simulink model "MultirotorModel"  (R2024b)
settings: Solver=VariableStepAuto  StartTime=0.0  StopTime=simTime  FixedStep=0.001  RelTol=1e-3  EnableMultiTasking=on
undefined symbols (not defined in the file): baseMission, bird_cycle, bird_end, bird_start, Controller, ctrl_mass, ctrl_thrust_perturbation_param, DiscIntNeverNeededParam, Dz, Earth, Gravity, initialConditions, Iz, mass_param, Nz, Pz, startFlightTime, UAVSampleTime, Vehicle, WGS84
libraries: slpidlib x10, uavalgslib x6, simulink x3, sharedutil x2, aerolibconvert2 x2, aerolibtransform2 x2, robotcorelib x1, uavutilslib x1, shared6dof x1, aerolibasang x1, sensorinslib x1
(part 1 of 3)
settings Model: DataDictionary=uavPackageDeliveryDataDict.sldd  ModifiedByFormat=The MathWorks, Inc.  SimulationMode=accelerator  PacingRate=3  Creator=The MathWorks, Inc.  LastModifiedBy=The MathWorks, Inc.
settings SolverCC: AlgebraicLoopSolver=TrustRegion  AutoInsertRateTranBlk=on  MaxZcPerStep=1
settings DataIOCC: LimitDataPoints=on  SaveOutput=off  SaveTime=off  ReturnWorkspaceOutputs=off
settings OptimizationCC: ReuseModelBlockBuffer=off  LifeSpan=inf
settings DebuggingCC: RTPrefix=none  SignalInfNanChecking=error  SignalRangeChecking=error  CheckMatrixSingularityMsg=error  ParameterPrecisionLossMsg=none  AllowSymbolicDim=off  SFUnexpectedBacktrackingDiag=warning  SFNoUnconditionalDefaultTransitionDiag=warning  SFExecutionAtInitializationDiag=none  ArithmeticOperatorsInVariantConditions=warning
settings ModelReferenceCC: EnableRefExpFcnMdlSchedulingChecks=on  PropagateSignalLabelsOutOfModel=off
settings SFSimCC: SimUseLocalCustomCode=off  CustomCodeUndefinedFunction=UseInterfaceOnly
settings RTWCC: RTWUseLocalCustomCode=off  GPUComputeCapability=3.5  DLArmComputeVersion=19.05
settings CodeAppCC: StateflowObjectComments=on
settings GRTTargetCC: TargetLangStandard=C89/C90 (ANSI)
settings ConfigComp: CovMetricSettings=dw  CovSaveCumulativeToWorkspaceVar=on  CovSaveSingleToWorkspaceVar=on  CovExternalEMLEnable=off

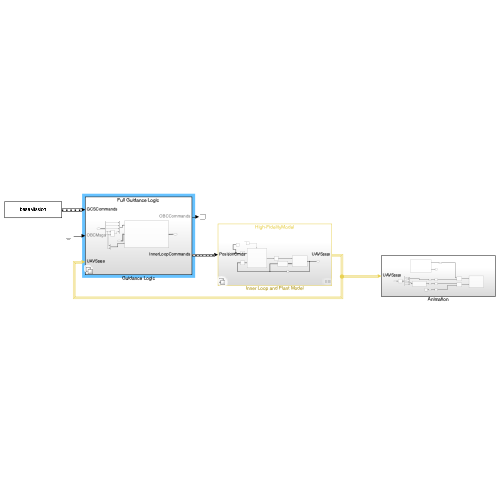
[thumbnail: Simulink's stored preview of the top-level diagram]
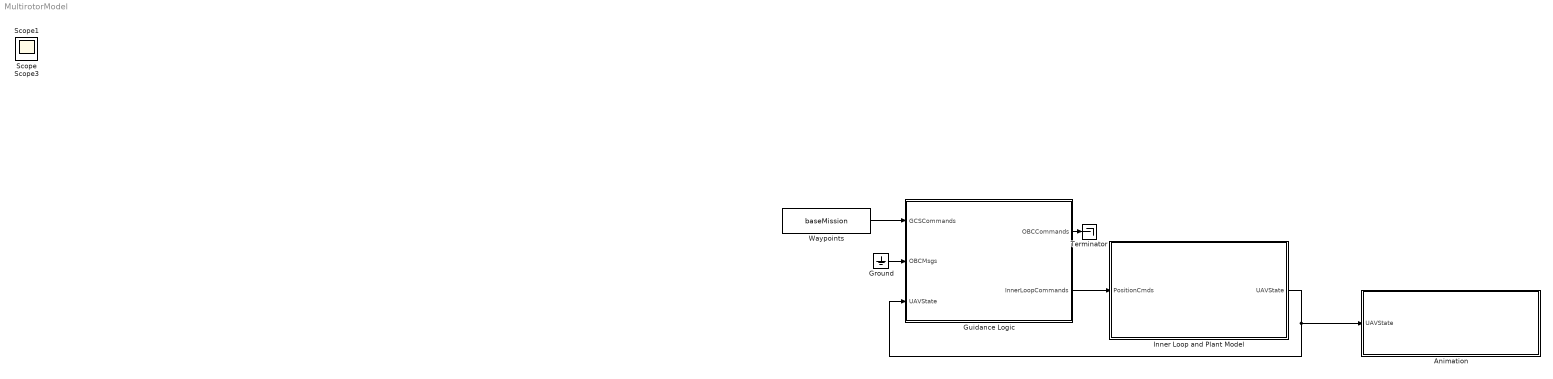
== system MultirotorModel ==
  Animation : Subsystem
  Ground : Ground
  Guidance Logic : Subsystem  Variant=on
  Inner Loop and Plant Model : Subsystem  Variant=on
  Terminator : Terminator
  Waypoints : Constant  Value=baseMission  OutDataTypeStr=Bus: uavPathManagerBus  SampleTime=-1
  Scope : Scope
  Scope1 : Scope
  Scope3 : Scope
  wires:
  Guidance Logic/2(InnerLoopCommands) -> Inner Loop and Plant Model/1(PositionCmds)
  Guidance Logic/1(OBCCommands) -> Terminator/1
  Ground/1 -> Guidance Logic/2(OBCMsgs)
  Waypoints/1 -> Guidance Logic/1(GCSCommands)
  Inner Loop and Plant Model/1(UAVState) -> Guidance Logic/3(UAVState), Animation/1(UAVState)

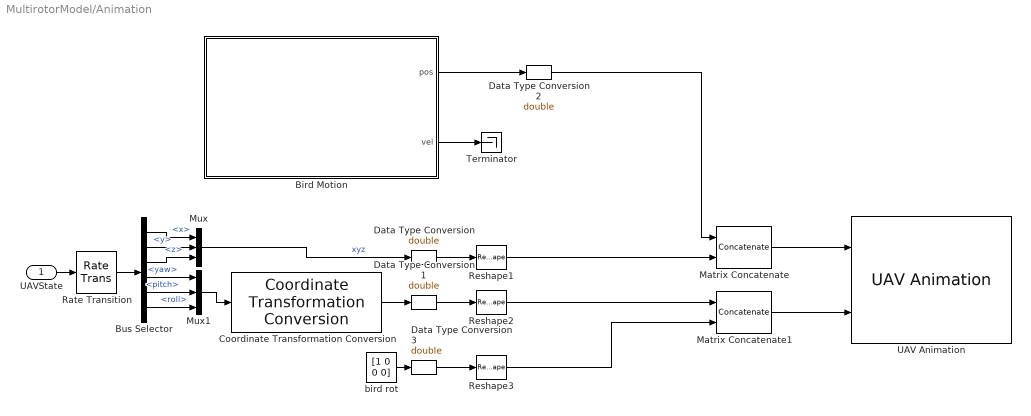
== system MultirotorModel/Animation ==
  UAVState : Inport
  Bird Motion : Subsystem
  Bus Selector : BusSelector  OutputSignals=pos_vel.x,pos_vel.y,pos_vel.z,attitude.yaw,attitude.pitch,attitude.roll
  Coordinate Transformation Conversion : robotcorelib/Coordinate Transformation Conversion  InputRepresentation=Euler Angles  InputEulerSequence=ZYX  ShowTrVecInputPort=on  OutputRepresentation=Quaternion  OutputEulerSequence=ZYX  ShowTrVecOutputPort=on  SimulateUsing=Code generation
  Data Type Conversion{,1..3} (4 alike) : DataTypeConversion  OutDataTypeStr=double  SaturateOnIntegerOverflow=off  RndMeth=Floor
  Matrix Concatenate : Concatenate  Mode=Multidimensional array
  Matrix Concatenate1 : Concatenate  Mode=Multidimensional array
  Mux : Mux  Inputs=3
  Mux1 : Mux  Inputs=3
  Rate Transition : RateTransition  OutPortSampleTime=UAVSampleTime*200
  Reshape1 : Reshape  OutputDimensionality=Row vector (2-D)
  Reshape2 : Reshape  OutputDimensionality=Row vector (2-D)
  Reshape3 : Reshape  OutputDimensionality=Row vector (2-D)
  Terminator : Terminator
  UAV Animation : uavutilslib/UAV Animation  NumUAV=2  DynamicUAVConfig=off  UAVType=Multirotor  UAVSize=1  UAVColor=[1 0 0]  UAVTrajectoryAlpha=1  InertialZDirection=Down  RotationFormat=Quaternion  DrawMarkers=off  SampleTime=UAVSampleTime*200
  bird rot : Constant  Value=[1 0 0 0]
  wires:
  Bus Selector/1 -> Mux/1  "<x>"
  Bus Selector/2 -> Mux/2  "<y>"
  Coordinate Transformation Conversion/1 -> Data Type Conversion1/1
  Rate Transition/1 -> Bus Selector/1
  Mux/1 -> Data Type Conversion/1  "xyz"
  UAVState/1 -> Rate Transition/1
  Bus Selector/6 -> Mux1/3  "<roll>"
  Bus Selector/4 -> Mux1/1  "<yaw>"
  Bus Selector/3 -> Mux/3  "<z>"
  Mux1/1 -> Coordinate Transformation Conversion/1
  Bus Selector/5 -> Mux1/2  "<pitch>"
  bird rot/1 -> Data Type Conversion3/1
  Data Type Conversion/1 -> Reshape1/1
  Data Type Conversion1/1 -> Reshape2/1
  Data Type Conversion3/1 -> Reshape3/1
  Data Type Conversion2/1 -> Matrix Concatenate/1
  Reshape1/1 -> Matrix Concatenate/2
  Matrix Concatenate/1 -> UAV Animation/1
  Reshape2/1 -> Matrix Concatenate1/1
  Reshape3/1 -> Matrix Concatenate1/2
  Matrix Concatenate1/1 -> UAV Animation/2
  Bird Motion/1(pos) -> Data Type Conversion2/1
  Bird Motion/2(vel) -> Terminator/1

== system MultirotorModel/Guidance Logic ==
  GCSCommands : Inport
  OBCMsgs : Inport  Port=2
  UAVState : Inport  Port=3
  Full Guidance Logic : Subsystem  TreatAsAtomicUnit=on  VariantControl=guidanceType==1
  Obstacle Avoidance : Subsystem  TreatAsAtomicUnit=on  SystemSampleTime=0.005*4  VariantControl=guidanceType ==2
  Obstacle Avoidance3D : Subsystem  TreatAsAtomicUnit=on  SystemSampleTime=0.005*4  VariantControl=guidanceType ==3
  OBCCommands : Outport  SampleTime=0.005  BusOutputAsStruct=on
  InnerLoopCommands : Outport  Port=2

== system MultirotorModel/Inner Loop and Plant Model ==
  PositionCmds : Inport
  High-FidelityModel : Subsystem  VariantControl=plantModelFi==1
  Low-FidelityModel : Subsystem  VariantControl=plantModelFi ==0
  UAVState : Outport

== system MultirotorModel/Animation/Bird Motion ==
  BirdMotion : MATLAB Function  TreatAsAtomicUnit=on
  Constant : Constant  Value=0.02
  Constant1 : Constant  Value=bird_start
  Constant2 : Constant  Value=bird_end
  Constant3 : Constant  Value=bird_cycle
  Demux : Demux  Outputs=6
  Mux : Mux  Inputs=3
  Mux1 : Mux  Inputs=3
  Reshape : Reshape  OutputDimensionality=Row vector (2-D)
  Sum : Sum  Inputs=|++
  Unit Delay : UnitDelay  SampleTime=0.02  HasFrameUpgradeWarning=on
  pos : Outport
  vel : Outport  Port=2
  wires:
  Unit Delay/1 -> Sum/2, BirdMotion/1(t)
  Sum/1 -> Unit Delay/1
  Constant/1 -> Sum/1
  Constant1/1 -> BirdMotion/2(start_pt)
  Constant2/1 -> BirdMotion/3(end_pt)
  Constant3/1 -> BirdMotion/4(cycle_time)
  BirdMotion/1(out) -> Demux/1
  Demux/1 -> Mux/1
  Demux/2 -> Mux/2
  Demux/3 -> Mux/3
  Demux/4 -> Mux1/1
  Demux/5 -> Mux1/2
  Demux/6 -> Mux1/3
  Mux/1 -> Reshape/1
  Mux1/1 -> vel/1
  Reshape/1 -> pos/1

== system MultirotorModel/Guidance Logic/Full Guidance Logic ==
  UAVState : Inport
  GCSCommands : Inport  Port=2
  Atan2 : Trigonometry  Operator=atan2
  Bus Selector1 : BusSelector  OutputSignals=pos_vel.x,pos_vel.y,pos_vel.z,pos_vel.vy,pos_vel.vx
  DroneVel : Mux  Inputs=2
  Guidance Stateflow : Subsystem
  Mux : Mux
  InnerLoopCommands : Outport
  wires:
  Mux/1 -> Guidance Stateflow/1(Pose)
  Bus Selector1/5 -> DroneVel/1, Atan2/2  "<vx>"
  Guidance Stateflow/1(InnerLoopCommands) -> InnerLoopCommands/1
  Bus Selector1/4 -> Atan2/1, DroneVel/2  "<vy>"
  Bus Selector1/3 -> Mux/3  "<z>"
  Bus Selector1/2 -> Mux/2  "<y>"
  UAVState/1 -> Bus Selector1/1
  Atan2/1 -> Mux/4
  Bus Selector1/1 -> Mux/1  "<x>"
  GCSCommands/1 -> Guidance Stateflow/2(GCSCommands)
  DroneVel/1 -> Guidance Stateflow/3(DroneVel)

== system MultirotorModel/Guidance Logic/Obstacle Avoidance ==
  GCSCommands : Inport
  OBCMsgs : Inport  Port=2
  UAVState : Inport  Port=3
  Bus Selector : BusSelector  OutputSignals=pos_vel
  Compute InnerLoop Cmds : Subsystem  TreatAsAtomicUnit=on
  MATLAB Function : MATLAB Function  TreatAsAtomicUnit=on
  Selector : Selector  InputPortWidth=42  IndexOptions=Index vector (dialog)  Indices=[1 2]  OutputSizes=1
  Unit Delay1 : UnitDelay  InitialCondition=single(0)  SampleTime=-1  HasFrameUpgradeWarning=on
  InnerLoopCommands : Outport
  OBCCommands : Outport  Port=2  BusOutputAsStruct=on
  wires:
  GCSCommands/1 -> Selector/1
  Unit Delay1/1 -> MATLAB Function/2(Steer)
  UAVState/1 -> Compute InnerLoop Cmds/2(UAVState), Bus Selector/1
  Bus Selector/1 -> MATLAB Function/3(UAVState)  "<pos_vel>"
  Selector/1 -> OBCCommands/1, MATLAB Function/1(mission)
  Compute InnerLoop Cmds/1(InnerLoopCmds) -> InnerLoopCommands/1
  MATLAB Function/1(y) -> Compute InnerLoop Cmds/1(GCSCmds)
  OBCMsgs/1 -> Unit Delay1/1

== system MultirotorModel/Guidance Logic/Obstacle Avoidance3D ==
  GCSCommands : Inport
  OBCMsgs : Inport  Port=2
  UAVState : Inport  Port=3
  Bus Selector : BusSelector  OutputSignals=pos_vel
  Compute InnerLoop Cmds : Subsystem  TreatAsAtomicUnit=on
  MATLAB Function : MATLAB Function  TreatAsAtomicUnit=on
  Selector : Selector  InputPortWidth=42  IndexOptions=Index vector (dialog)  Indices=[1 2]  OutputSizes=1
  Unit Delay1 : UnitDelay  InitialCondition=single(0)  SampleTime=-1  HasFrameUpgradeWarning=on
  InnerLoopCommands : Outport
  OBCCommands : Outport  Port=2  BusOutputAsStruct=on
  wires:
  MATLAB Function/1(y) -> Compute InnerLoop Cmds/1(GCSCmds)
  Unit Delay1/1 -> MATLAB Function/2(Steer)
  Selector/1 -> MATLAB Function/1(mission), OBCCommands/1
  Bus Selector/1 -> MATLAB Function/3(UAVState)  "<pos_vel>"
  GCSCommands/1 -> Selector/1
  OBCMsgs/1 -> Unit Delay1/1
  MATLAB Function/2(DTD) -> Compute InnerLoop Cmds/2(DTD)
  Compute InnerLoop Cmds/1(InnerLoopCmds) -> InnerLoopCommands/1
  UAVState/1 -> Bus Selector/1, Compute InnerLoop Cmds/4(UAVState)
  MATLAB Function/3(needHover) -> Compute InnerLoop Cmds/3(needHover)

== system MultirotorModel/Inner Loop and Plant Model/High-FidelityModel ==
  note: To be replaced with a signal from the GCS to "Start Mission"
  PositionCmds : Inport
  Control System : Subsystem  TreatAsAtomicUnit=on  SystemSampleTime=UAVSampleTime
  Environment : Subsystem  TreatAsAtomicUnit=on  VariantControl=VSS_ENVIRONMENT_VARIABLE
  Memory1 : Memory  InheritSampleTime=on  LinearizeMemory=on  LinearizeAsDelay=on
  Plant Model : Subsystem  TreatAsAtomicUnit=on
  Rate Transition : RateTransition
  Rate Transition1 : RateTransition  OutPortSampleTime=UAVSampleTime
  Rate Transition2 : RateTransition  OutPortSampleTime=UAVSampleTime
  Scope : Scope
  Step : Step  Time=startFlightTime  SampleTime=UAVSampleTime
  UAVState : Outport  OutDataTypeStr=Bus: uavStateBus
  wires:
  PositionCmds/1 -> Scope/1, Rate Transition1/1
  Control System/1(ActuatorCmds) -> Rate Transition/1  "motors"
  Environment/1(Environment) -> Plant Model/2(Environment)
  Memory1/1 -> Environment/1(States), Rate Transition2/1
  Plant Model/1(UAVState) -> UAVState/1, Memory1/1
  Step/1 -> Control System/Enable
  Rate Transition/1 -> Plant Model/1(Actuators)
  Rate Transition1/1 -> Control System/1(PositionCmd)
  Rate Transition2/1 -> Control System/2(UAVState)

== system MultirotorModel/Inner Loop and Plant Model/Low-FidelityModel ==
  PositionCmds : Inport
  Assemble UAV State Bus : Subsystem
  Bus Creator1 : BusCreator  Inputs=1  OutDataTypeStr=Bus: uavGuidanceEnvironmentBus  NonVirtualBus=on
  Constant : Constant  Value=Gravity  OutDataTypeStr=single
      settings: AttributesFormatString=%<Value>
  Position and Acceleration Control : Subsystem
  Quadrotor Plant : uavalgslib/Guidance Model  ModelType=MultirotorGuidance  SpecifiedDataType=single  SimulateUsing=Code generation  InitialWorldPositionMultirotor=[-186; -105; 0]  InitialWorldVelocityMultirotor=[0; 0; 0]  InitialEulerZYXMultirotor=[0; 0; 0]  InitialBodyAngularRateRPYMultirotor=[0; 0; 0]  InitialThrustMultirotor=0  InitialNorthFixedWing=0  InitialEastFixedWing=0  InitialHeightFixedWing=0  InitialAirSpeedFixedWing=0  InitialHeadingAngleFixedWing=0  InitialFlightPathAngleFixedWing=0  InitialRollAngleFixedWing=0  InitialRollAngleRateFixedWing=0  PDRollMultirotor=[3402.97,116.67]  PDPitchMultirotor=[3402.97, 116.67]  PYawRateMultirotor=1950  PThrustMultirotor=39  MassMultirotor=0.1  PHeightFixedWing=3.9  PHeadingAngleFixedWing=3.9  PFlightPathAngleFixedWing=39  PDRollFixedWing=[3402.97, 116.67]  PAirSpeedFixedWing=1  FlightPathAngleLimitsFixedWing=[-pi/2, pi/2]  StateBusName='uavGuidanceStateBus'  ControlBusName='uavGuidanceControlBus'  EnvironmentBusName='uavGuidanceEnvironmentBus'  DataType=single
  Rate Transition1 : RateTransition  OutPortSampleTime=UAVSampleTime
  Rate Transition2 : RateTransition  OutPortSampleTime=UAVSampleTime
  UAVState : Outport  OutDataTypeStr=Bus: uavStateBus
  wires:
  Constant/1 -> Bus Creator1/1  "Gravity"
  Bus Creator1/1 -> Quadrotor Plant/2
  Position and Acceleration Control/1(Control Signal) -> Rate Transition2/1
  Quadrotor Plant/1 -> Rate Transition1/1
  Rate Transition2/1 -> Quadrotor Plant/1
  PositionCmds/1 -> Position and Acceleration Control/2(PositionCmd)
  Rate Transition1/1 -> Position and Acceleration Control/1(QuadRotorState), Assemble UAV State Bus/1(State)
  Assemble UAV State Bus/1(UAVState) -> UAVState/1

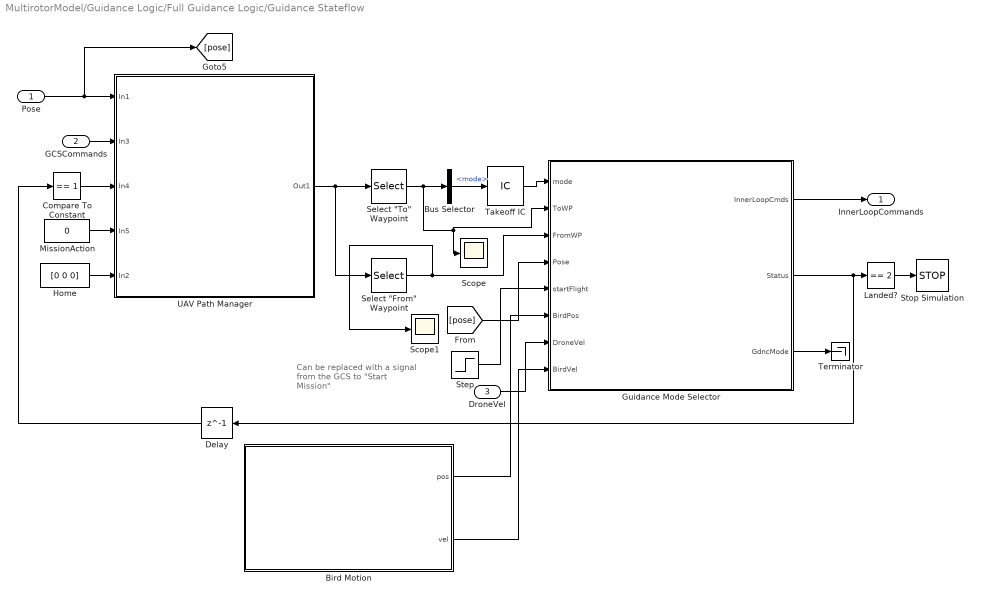
== system MultirotorModel/Guidance Logic/Full Guidance Logic/Guidance Stateflow ==
  note: Can be replaced with a signal from the GCS to "Start Mission"
  Pose : Inport
  GCSCommands : Inport  Port=2
  DroneVel : Inport  Port=3
  Bird Motion : Subsystem
  Bus Selector : BusSelector  OutputSignals=mode
  Compare To Constant : simulink/Logic and Bit Operations/Compare To Constant  relop===  const=1  OutDataTypeStr=boolean
  Delay : Delay  DelayLength=1  InitialCondition=0
  Guidance Mode Selector : Stateflow chart  TreatAsAtomicUnit=on
  Home : Constant  Value=[0 0 0]  OutDataTypeStr=single
  Landed? : simulink/Logic and Bit Operations/Compare To Constant  relop===  const=2  OutDataTypeStr=boolean
  MissionAction : Constant  Value=0  OutDataTypeStr=uint8
  Scope : Scope
  Scope1 : Scope
  "Select \"From\" Waypoint" : Selector  InputPortWidth=2  IndexOptions=Index vector (dialog)  Indices=2  OutputSizes=1
  "Select \"To\" Waypoint" : Selector  InputPortWidth=2  IndexOptions=Index vector (dialog)  Indices=1  OutputSizes=1
  Step : Step  Time=startFlightTime  SampleTime=UAVSampleTime*4
  Stop Simulation : Stop
  Takeoff IC : InitialCondition
  Terminator : Terminator
  UAV Path Manager : Subsystem  AncestorBlock=uavalgslib/Path Manager  mask(Path Manager){UAVType=multirotor, LoiterRadius=25, dataType=single, inputBusName='uavPathManagerBus', SimulateUsing=Code generation}
      mask prompts: UAVType "uav:robotsluav:pathmanager:UAVType"; LoiterRadius "uav:robotsluav:pathmanager:LoiterRadius"; dataType "uav:robotsluav:pathmanager:DataType"; inputBusName "uav:robotsluav:pathmanager:InputBusName"; SimulateUsing "SystemBlock:MATLABSystem:SimulateUsing"
      mask help: uav:robotsluav:pathmanager:PathManagerDescription
      mask Help: eval('helpview(''uav'',''uavPathManager'')');
      mask TypeOptions UAVType: PathManagerSystemObject/UAVType
      mask Callback UAVType: uav.sluav.internal.pathmanager.mask.setLoiterParameter(gcb);
      mask TypeOptions LoiterRadius: PathManagerSystemObject/LoiterRadius
      mask Callback dataType:
      | if ~strcmp(get_param(gcb, 'dataType'), '<data type expression>')
      | 
      |     %create path manager bus
      |     uav.sluav.internal.pathmanager.mask.createUAVPathManagerBus(gcb);
      | 
      | end
      mask Callback inputBusName: uav.sluav.internal.pathmanager.mask.createUAVPathManagerBus(gcb);
      mask TypeOptions SimulateUsing: PathManagerSystemObject/SimulateUsing
      mask DialogControl UAVType Prompt: UAV type:
      mask DialogControl LoiterRadius Prompt: Loiter radius (m):
      mask DialogControl dataType Prompt: Data type:
      mask DialogControl inputBusName Prompt: Mission bus name:
      mask DialogControl SimulateUsing Prompt: Simulate using:
      mask Display:
      | port_label('input',1,'Pose')
      | port_label('input',2,'MissionData')
      | port_label('input',3,'isModeDone')
      | port_label('input',4,'MissionCmd')
      | port_label('input',5,'Home')
      | port_label('output',1,'MissionParams')
  InnerLoopCommands : Outport  OutDataTypeStr=Bus: innerLoopCmdsBus
  wires:
  Takeoff IC/1 -> Guidance Mode Selector/1(mode)
  Delay/1 -> Compare To Constant/1
  Guidance Mode Selector/2(Status) -> Delay/1, Landed?/1
  Guidance Mode Selector/1(InnerLoopCmds) -> InnerLoopCommands/1
  Pose/1 -> UAV Path Manager/1(In1), [pose]
  UAV Path Manager/1(Out1) -> "Select \"From\" Waypoint"/1, "Select \"To\" Waypoint"/1
  Bus Selector/1 -> Takeoff IC/1  "<mode>"
  [pose] -> Guidance Mode Selector/4(Pose)
  "Select \"To\" Waypoint"/1 -> Scope/1, Guidance Mode Selector/2(ToWP), Bus Selector/1
  "Select \"From\" Waypoint"/1 -> Scope1/1, Guidance Mode Selector/3(FromWP)
  Landed?/1 -> Stop Simulation/1
  Step/1 -> Guidance Mode Selector/5(startFlight)
  Guidance Mode Selector/3(GdncMode) -> Terminator/1
  Home/1 -> UAV Path Manager/5(In2)
  MissionAction/1 -> UAV Path Manager/4(In5)
  Compare To Constant/1 -> UAV Path Manager/3(In4)
  GCSCommands/1 -> UAV Path Manager/2(In3)
  Bird Motion/1(pos) -> Guidance Mode Selector/6(BirdPos)
  DroneVel/1 -> Guidance Mode Selector/7(DroneVel)
  Bird Motion/2(vel) -> Guidance Mode Selector/8(BirdVel)

== system MultirotorModel/Guidance Logic/Obstacle Avoidance/Compute InnerLoop Cmds ==
  GCSCmds : Inport
  UAVState : Inport  Port=2
  Atan2 : Trigonometry  Operator=atan2
  Bus Creator : BusCreator  Inputs=3  OutDataTypeStr=Bus: innerLoopCmdsBus  NonVirtualBus=on
  Bus Selector1 : BusSelector  OutputSignals=pos_vel.x,pos_vel.y,pos_vel.z,pos_vel.vy,pos_vel.vx
  Lookahead Distance : Constant  Value=5  OutDataTypeStr=single
  Mux : Mux
  Scope : Scope
  Scope1 : Scope
  Terminator : Terminator
  Waypoint Follower : uavalgslib/Waypoint Follower  UAVType=multirotor  StartFrom=first  TransitionRadiusSource=internal  TransitionRadius=0.5  MinLookaheadDistance=0.1  HoverAtLastWaypoint=off  YawInput=on  ShowCrossTrackErrorOutput=on  ShowStatusOutput=on  SimulateUsing=Code generation
  InnerLoopCmds : Outport  OutDataTypeStr=Bus: innerLoopCmdsBus
  wires:
  Atan2/1 -> Mux/4
  Lookahead Distance/1 -> Waypoint Follower/3
  UAVState/1 -> Bus Selector1/1
  Bus Selector1/2 -> Mux/2  "<y>"
  Bus Selector1/1 -> Mux/1  "<x>"
  Bus Selector1/4 -> Atan2/1  "<vy>"
  Mux/1 -> Waypoint Follower/1
  Bus Selector1/5 -> Atan2/2  "<vx>"
  Bus Selector1/3 -> Mux/3  "<z>"
  Bus Creator/1 -> InnerLoopCmds/1
  Waypoint Follower/1 -> Bus Creator/1  "LAP"
  Waypoint Follower/2 -> Bus Creator/2  "HeadingCmd"
  Waypoint Follower/3 -> Bus Creator/3  "YawCmd"
  GCSCmds/1 -> Waypoint Follower/2
  Waypoint Follower/5 -> Scope/1
  Waypoint Follower/4 -> Terminator/1
  Waypoint Follower/6 -> Scope1/1

== system MultirotorModel/Guidance Logic/Obstacle Avoidance3D/Compute InnerLoop Cmds ==
  GCSCmds : Inport
  DTD : Inport  Port=2
  needHover : Inport  Port=3
  UAVState : Inport  Port=4
  FollowWaypoints : Subsystem
  GCSCmds1 : InportShadow
  GCSCmds2 : InportShadow
  Hover : Subsystem
  Landing : Subsystem
  Switch1 : Switch  Threshold=5  SaturateOnIntegerOverflow=off  InputSameDT=off
  Switch2 : Switch  Criteria=u2 ~= 0  Threshold=5  SaturateOnIntegerOverflow=off  InputSameDT=off
  UAVState1 : InportShadow  Port=4
  InnerLoopCmds : Outport  OutDataTypeStr=Bus: innerLoopCmdsBus
  wires:
  Switch2/1 -> InnerLoopCmds/1
  GCSCmds2/1 -> Hover/1(In1)
  UAVState1/1 -> Landing/2(UAVState1)
  Hover/1(Out1) -> Switch2/1
  Landing/1(InnerLoopCmds1) -> Switch1/3
  Switch1/1 -> Switch2/3
  GCSCmds1/1 -> Landing/1(GCSCmds)
  FollowWaypoints/1(InnerLoopCmds) -> Switch1/1
  DTD/1 -> Switch1/2
  UAVState/1 -> FollowWaypoints/1(UAVState)
  GCSCmds/1 -> FollowWaypoints/2(GCSCmds)
  needHover/1 -> Switch2/2

== system MultirotorModel/Inner Loop and Plant Model/High-FidelityModel/Control System ==
  PositionCmd : Inport
  UAVState : Inport  Port=2  BusOutputAsStruct=on
  Enable : EnablePort  StatesWhenEnabling=reset
  Controller : Subsystem
  ActuatorCmds : Outport  VectorParamsAs1DForOutWhenUnconnected=off
  wires:
  Controller/1(motors_refout) -> ActuatorCmds/1
  UAVState/1 -> Controller/2(UAVState)
  PositionCmd/1 -> Controller/1(PositionCmd)

== system MultirotorModel/Inner Loop and Plant Model/High-FidelityModel/Environment ==
  States : Inport
  Bus Creator : BusCreator  Inputs=3  OutDataTypeStr=Bus: EnvironmentBus  NonVirtualBus=on
  Bus Creator1 : BusCreator  Inputs=4  OutDataTypeStr=Bus: AtmosphereBus  NonVirtualBus=on
  Bus Selector : BusSelector  OutputSignals=gps.lat,gps.lon,gps.alt
  Constant : Constant  Value=288.08
  Constant1 : Constant  Value=340.25
  Constant2 : Constant  Value=1.012*10^5
  Constant3 : Constant  Value=1.224
  Gain : Gain  Gain=1/1e7  OutDataTypeStr=double
  Gain1 : Gain  Gain=1/1e7  OutDataTypeStr=double
  Gain2 : Gain  Gain=1/-1e3  OutDataTypeStr=double
  Magnetic feild : Constant  Value=[19080, -1276, 50282]
  Mux : Mux  Inputs=3
  "WGS84 Gravity Model  " : GravityWGS84  action=None
  Environment : Outport  VectorParamsAs1DForOutWhenUnconnected=off
  wires:
  States/1 -> Bus Selector/1  "StatesLog"
  Bus Creator/1 -> Environment/1
  Bus Creator1/1 -> Bus Creator/2  "AtmosphereBus"
  "WGS84 Gravity Model  "/1 -> Bus Creator/1  "Gravity_ned"
  Mux/1 -> "WGS84 Gravity Model  "/1
  Gain/1 -> Mux/1
  Bus Selector/1 -> Gain/1  "<lat>"
  Bus Selector/2 -> Gain1/1  "<lon>"
  Gain1/1 -> Mux/2
  Bus Selector/3 -> Gain2/1  "<alt>"
  Gain2/1 -> Mux/3
  Magnetic feild/1 -> Bus Creator/3  "MagneticField_ned"
  Constant/1 -> Bus Creator1/1  "air_temp"
  Constant1/1 -> Bus Creator1/2  "speed_sound"
  Constant2/1 -> Bus Creator1/3  "pressure"
  Constant3/1 -> Bus Creator1/4  "air_density"

== system MultirotorModel/Inner Loop and Plant Model/High-FidelityModel/Plant Model ==
  Actuators : Inport
  Environment : Inport  Port=2
  6DOF (Quaternion) : shared6dof/6DOF (Euler Angles)  units=Metric (MKS)  mtype=Fixed  rep=Euler Angles  xme_0=initialConditions.posNED + [0 0 -1]  Vm_0=[0 0 0]  eul_0=[0,0,0]  pm_0=[0,0,0]  mass_0=mass_param  mass_e=0.5  mass_f=2.0  inertia=Vehicle.Airframe.inertia  inertia_e=eye(3)  inertia_f=2*eye(3)  k_quat=Vehicle.SixDOF.quatGain  vre_flag=on  abi_flag=on  aMode=aMode  xme_statename=''  Vm_statename=''  eul_statename=''  quat_statename=''  pm_statename=''  mass_statename=''
  AC model : Subsystem
  Bus setup : Subsystem
  IMU Drift : FromWorkspace  VariableName=gyro_drift_signal  SampleTime=0.1
  Scope : Scope
  Sum1 : Sum  Inputs=|++
  Terminator1 : Terminator
  Terminator2 : Terminator
  Terminator3 : Terminator
  UAVState : Outport  VectorParamsAs1DForOutWhenUnconnected=off
  wires:
  Actuators/1 -> AC model/1(Actuators)
  Environment/1 -> AC model/2(Environment)
  6DOF (Quaternion)/1 -> Bus setup/1(V_ned)
  6DOF (Quaternion)/2 -> Bus setup/2(X_ned), Scope/1  "X_e"
  6DOF (Quaternion)/6 -> Bus setup/5(Omega_b), AC model/5(w_b)
  6DOF (Quaternion)/4 -> Bus setup/4(DCM), AC model/3(DCM_be)
  Bus setup/1(UAVState) -> UAVState/1
  6DOF (Quaternion)/7 -> Terminator2/1
  6DOF (Quaternion)/8 -> Terminator3/1
  AC model/1(F_cg) -> 6DOF (Quaternion)/1
  AC model/2(M_cg) -> 6DOF (Quaternion)/2
  6DOF (Quaternion)/5 -> AC model/4(V_b)
  6DOF (Quaternion)/3 -> Sum1/1
  Sum1/1 -> Bus setup/3(Euler)
  IMU Drift/1 -> Sum1/2
  6DOF (Quaternion)/9 -> Terminator1/1

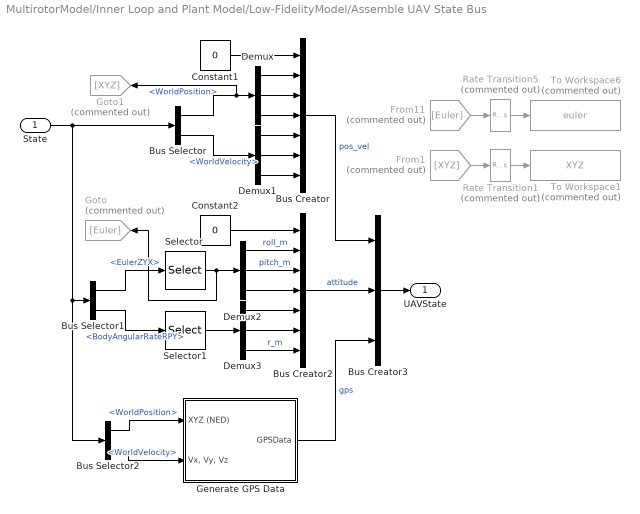
== system MultirotorModel/Inner Loop and Plant Model/Low-FidelityModel/Assemble UAV State Bus ==
  State : Inport
  Bus Creator : BusCreator  Inputs=7  OutDataTypeStr=Bus: local_position_ned
      settings: InheritFromInputs=off
  Bus Creator2 : BusCreator  Inputs=7  OutDataTypeStr=Bus: attitudeBus
      settings: InheritFromInputs=off
  Bus Creator3 : BusCreator  Inputs=3  OutDataTypeStr=Bus: uavStateBus
      settings: InheritFromInputs=off
  Bus Selector : BusSelector  OutputSignals=WorldPosition,WorldVelocity
  Bus Selector1 : BusSelector  OutputSignals=EulerZYX,BodyAngularRateRPY
  Bus Selector2 : BusSelector  OutputSignals=WorldPosition,WorldVelocity
  Constant1 : Constant  Value=0  OutDataTypeStr=uint32
  Constant2 : Constant  Value=0  OutDataTypeStr=uint32
  Demux{,1..3} (4 alike) : Demux  Outputs=3
  From1 : From  Commented=on  GotoTag=XYZ
  From11 : From  Commented=on  GotoTag=Euler
  Generate GPS Data : Subsystem
  Goto : Goto  Commented=on  GotoTag=Euler
  Goto1 : Goto  Commented=on  GotoTag=XYZ
  Rate Transition1 : RateTransition  Commented=on  OutPortSampleTime=UAVSampleTime
  Rate Transition5 : RateTransition  Commented=on  OutPortSampleTime=UAVSampleTime
  Selector : Selector  InputPortWidth=3  IndexOptions=Index vector (dialog)  Indices=[3 2 1]  OutputSizes=1
  Selector1 : Selector  InputPortWidth=3  IndexOptions=Index vector (dialog)  Indices=[3 2 1]  OutputSizes=1
  To Workspace1 : ToWorkspace  Commented=on  VariableName=XYZ  SaveFormat=Timeseries  SampleTime=-1
  To Workspace6 : ToWorkspace  Commented=on  VariableName=euler  SaveFormat=Timeseries  SampleTime=-1
  UAVState : Outport  OutDataTypeStr=Bus: uavStateBus
  wires:
  Bus Creator2/1 -> Bus Creator3/2  "attitude"
  Bus Creator3/1 -> UAVState/1
  Demux3/1 -> Bus Creator2/5
  Demux1/2 -> Bus Creator/6
  Bus Creator/1 -> Bus Creator3/1  "pos_vel"
  Demux1/3 -> Bus Creator/7
  Bus Selector2/2 -> Generate GPS Data/2("Vx, Vy, Vz")  "<WorldVelocity>"
  Demux/1 -> Bus Creator/2
  State/1 -> Bus Selector/1, Bus Selector2/1, Bus Selector1/1
  Constant2/1 -> Bus Creator2/1
  Bus Selector/1 -> Goto1/1, Demux/1  "<WorldPosition>"
  Selector1/1 -> Demux3/1
  Demux1/1 -> Bus Creator/5
  Bus Selector1/1 -> Selector/1  "<EulerZYX>"
  Demux/2 -> Bus Creator/3
  Demux2/1 -> Bus Creator2/2  "roll_m"
  Demux2/3 -> Bus Creator2/4
  Demux3/2 -> Bus Creator2/6
  Demux2/2 -> Bus Creator2/3  "pitch_m"
  Bus Selector1/2 -> Selector1/1  "<BodyAngularRateRPY>"
  Demux3/3 -> Bus Creator2/7  "r_m"
  Demux/3 -> Bus Creator/4
  Bus Selector/2 -> Demux1/1  "<WorldVelocity>"
  Constant1/1 -> Bus Creator/1
  Bus Selector2/1 -> Generate GPS Data/1(XYZ (NED))  "<WorldPosition>"
  Generate GPS Data/1(GPSData) -> Bus Creator3/3  "gps"
  Rate Transition5/1 -> To Workspace6/1
  From11/1 -> Rate Transition5/1
  Selector/1 -> Goto/1, Demux2/1
  From1/1 -> Rate Transition1/1
  Rate Transition1/1 -> To Workspace1/1

== system MultirotorModel/Inner Loop and Plant Model/Low-FidelityModel/Position and Acceleration Control ==
  note: To be replaced with a signal from the GCS to "Start Mission"
  QuadRotorState : Inport
  PositionCmd : Inport  Port=2
  Attitude Control : Subsystem
  Position Control : Subsystem
  Step : Step  Time=startFlightTime  SampleTime=UAVSampleTime
  Velocity Control : Subsystem
  Control Signal : Outport
  wires:
  PositionCmd/1 -> Position Control/1(PositionCmd), Attitude Control/3(PositionCmd)
  Velocity Control/1(Accel Cmd) -> Attitude Control/1(Accel Cmd)
  Attitude Control/1(Control Signal) -> Control Signal/1
  QuadRotorState/1 -> Velocity Control/2(QuadRotorState), Attitude Control/2(QuadRotorState), Position Control/2(QuadRotorState)
  Position Control/1(Velocity Cmd) -> Velocity Control/1(Velocity Cmd)
  Step/1 -> Velocity Control/Enable, Position Control/Enable

== system MultirotorModel/Guidance Logic/Full Guidance Logic/Guidance Stateflow/Bird Motion ==
  BirdMotion : MATLAB Function  TreatAsAtomicUnit=on
  Constant : Constant  Value=0.02
  Constant1 : Constant  Value=bird_start
  Constant2 : Constant  Value=bird_end
  Constant3 : Constant  Value=bird_cycle
  Demux : Demux  Outputs=6
  Mux : Mux  Inputs=3
  Mux1 : Mux  Inputs=3
  Reshape : Reshape  OutputDimensionality=Row vector (2-D)
  Sum : Sum  Inputs=|++
  Unit Delay : UnitDelay  SampleTime=0.02  HasFrameUpgradeWarning=on
  pos : Outport
  vel : Outport  Port=2
  wires:
  Unit Delay/1 -> Sum/2, BirdMotion/1(t)
  Sum/1 -> Unit Delay/1
  Constant/1 -> Sum/1
  Constant1/1 -> BirdMotion/2(start_pt)
  Constant2/1 -> BirdMotion/3(end_pt)
  Constant3/1 -> BirdMotion/4(cycle_time)
  BirdMotion/1(out) -> Demux/1
  Demux/1 -> Mux/1
  Demux/2 -> Mux/2
  Demux/3 -> Mux/3
  Demux/4 -> Mux1/1
  Demux/5 -> Mux1/2
  Demux/6 -> Mux1/3
  Mux/1 -> Reshape/1
  Mux1/1 -> vel/1
  Reshape/1 -> pos/1

== system MultirotorModel/Guidance Logic/Full Guidance Logic/Guidance Stateflow/Guidance Mode Selector/GuidanceLogic.Land.Descend ==
  ToWP : Inport
  Action Port : ActionPort
      settings: CopyFcn=Stateflow.SLINSF.SimulinkMan.removeBlockPreDeleteFcn  PreDeleteFcn=Stateflow.SLINSF.SimulinkMan.unsafePredeleteFcn
  Bus Creator : BusCreator  Inputs=3  OutDataTypeStr=Bus: innerLoopCmdsBus  NonVirtualBus=on
      settings: InheritFromInputs=off
  Bus Selector : BusSelector  OutputSignals=position,params
  Demux1 : Demux  Outputs=[2 1]
  Hdg Cmd Sat : Saturate  UpperLimit=pi  LowerLimit=-pi
      settings: AttributesFormatString=[%<UpperLimit> %<LowerLimit>]
  Mux : Mux  Inputs=2
  Selector1 : Selector  InputPortWidth=4  IndexOptions=Index vector (dialog)  Indices=4  OutputSizes=1
  Selector3 : Selector  InputPortWidth=4  IndexOptions=Index vector (dialog)  Indices=4  OutputSizes=1
  Yaw Cmd Sat : Saturate  UpperLimit=pi  LowerLimit=-pi
      settings: AttributesFormatString=[%<UpperLimit> %<LowerLimit>]
  InnerLoopCmds : Outport  OutDataTypeStr=Bus: innerLoopCmdsBus
  wires:
  Bus Creator/1 -> InnerLoopCmds/1
  Mux/1 -> Bus Creator/1  "LAP"
  Bus Selector/2 -> Selector1/1, Selector3/1  "<params>"
  Bus Selector/1 -> Demux1/1  "<position>"
  Yaw Cmd Sat/1 -> Bus Creator/3  "YawCmd"
  Hdg Cmd Sat/1 -> Bus Creator/2  "HeadingCmd"
  ToWP/1 -> Bus Selector/1
  Demux1/2 -> Mux/2
  Demux1/1 -> Mux/1
  Selector1/1 -> Yaw Cmd Sat/1
  Selector3/1 -> Hdg Cmd Sat/1

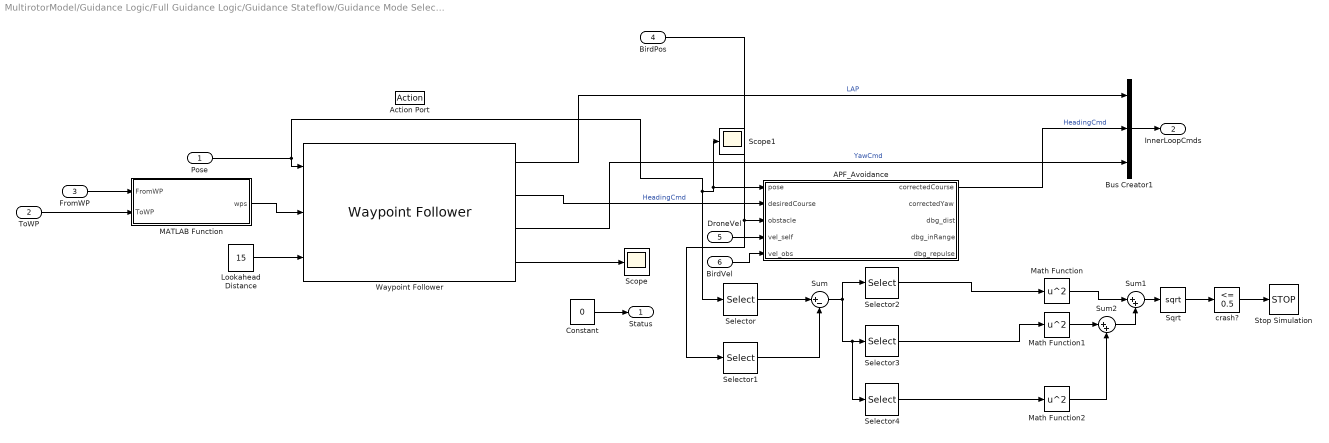
== system MultirotorModel/Guidance Logic/Full Guidance Logic/Guidance Stateflow/Guidance Mode Selector/GuidanceLogic.Land.ToLand ==
  Pose : Inport
  ToWP : Inport  Port=2
  FromWP : Inport  Port=3
  "BirdPos " : Inport  Port=4
  DroneVel : Inport  Port=5
  BirdVel : Inport  Port=6
  Action Port : ActionPort
      settings: CopyFcn=Stateflow.SLINSF.SimulinkMan.removeBlockPreDeleteFcn  PreDeleteFcn=Stateflow.SLINSF.SimulinkMan.unsafePredeleteFcn
  APF_Avoidance : MATLAB Function  TreatAsAtomicUnit=on
  Bus Creator1 : BusCreator  Inputs=3  OutDataTypeStr=Bus: innerLoopCmdsBus  NonVirtualBus=on
  Constant : Constant  Value=0  OutDataTypeStr=uint8
  Lookahead Distance : Constant  Value=15  OutDataTypeStr=single
  MATLAB Function : MATLAB Function  TreatAsAtomicUnit=on
  Math Function : Math  Operator=square
  Math Function1 : Math  Operator=square
  Math Function2 : Math  Operator=square
  Scope : Scope
  Scope1 : Scope
  Selector : Selector  InputPortWidth=4  IndexOptions=Index vector (dialog)  Indices=[1 2 3]  OutputSizes=1
  Selector1 : Selector  InputPortWidth=3  IndexOptions=Index vector (dialog)  Indices=[1 2 3]  OutputSizes=1
  Selector2 : Selector  InputPortWidth=3  IndexOptions=Index vector (dialog)  Indices=[1]  OutputSizes=1
  Selector3 : Selector  InputPortWidth=3  IndexOptions=Index vector (dialog)  Indices=[2]  OutputSizes=1
  Selector4 : Selector  InputPortWidth=3  IndexOptions=Index vector (dialog)  Indices=[3]  OutputSizes=1
  Sqrt : Sqrt
  Stop Simulation : Stop
  Sum : Sum  Inputs=|+-
  Sum1 : Sum  Inputs=|++
  Sum2 : Sum  Inputs=|++
  Waypoint Follower : uavalgslib/Waypoint Follower  UAVType=multirotor  StartFrom=closest  TransitionRadiusSource=internal  TransitionRadius=10  MinLookaheadDistance=0.1  HoverAtLastWaypoint=off  YawInput=on  ShowCrossTrackErrorOutput=off  ShowStatusOutput=off  SimulateUsing=Code generation
  crash? : simulink/Logic and Bit Operations/Compare To Constant  relop=<=  const=0.5  OutDataTypeStr=boolean
  Status : Outport
  InnerLoopCmds : Outport  Port=2  OutDataTypeStr=Bus: innerLoopCmdsBus
  wires:
  Constant/1 -> Status/1
  MATLAB Function/1(wps) -> Waypoint Follower/2
  Lookahead Distance/1 -> Waypoint Follower/3
  Waypoint Follower/1 -> Bus Creator1/1  "LAP"
  Bus Creator1/1 -> InnerLoopCmds/1
  Waypoint Follower/2 -> APF_Avoidance/2(desiredCourse)  "HeadingCmd"
  FromWP/1 -> MATLAB Function/1(FromWP)
  Waypoint Follower/4 -> Scope/1
  Pose/1 -> Scope1/1, APF_Avoidance/1(pose), Selector/1, Waypoint Follower/1
  APF_Avoidance/1(correctedCourse) -> Bus Creator1/2  "HeadingCmd"
  Selector/1 -> Sum/1
  Selector1/1 -> Sum/2
  Sqrt/1 -> crash?/1
  crash?/1 -> Stop Simulation/1
  Selector2/1 -> Math Function/1
  Selector3/1 -> Math Function1/1
  Sum1/1 -> Sqrt/1
  Math Function/1 -> Sum1/1
  Sum/1 -> Selector4/1, Selector3/1, Selector2/1
  Math Function1/1 -> Sum2/1
  Sum2/1 -> Sum1/2
  Selector4/1 -> Math Function2/1
  Math Function2/1 -> Sum2/2
  "BirdPos "/1 -> Selector1/1, APF_Avoidance/3(obstacle)
  ToWP/1 -> MATLAB Function/2(ToWP)
  Waypoint Follower/3 -> Bus Creator1/3  "YawCmd"
  DroneVel/1 -> APF_Avoidance/4(vel_self)
  BirdVel/1 -> APF_Avoidance/5(vel_obs)

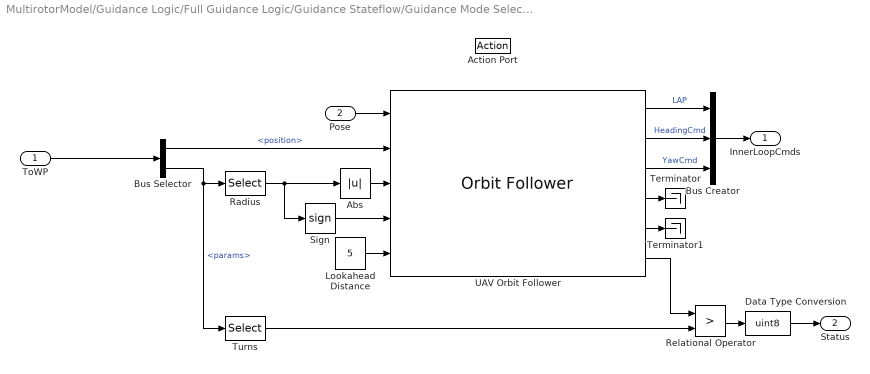
== system MultirotorModel/Guidance Logic/Full Guidance Logic/Guidance Stateflow/Guidance Mode Selector/GuidanceLogic.Orbit ==
  ToWP : Inport
  Pose : Inport  Port=2
  Action Port : ActionPort
      settings: CopyFcn=Stateflow.SLINSF.SimulinkMan.removeBlockPreDeleteFcn  PreDeleteFcn=Stateflow.SLINSF.SimulinkMan.unsafePredeleteFcn
  Abs : Abs  SaturateOnIntegerOverflow=off
  Bus Creator : BusCreator  Inputs=3  OutDataTypeStr=Bus: innerLoopCmdsBus  NonVirtualBus=on
  Bus Selector : BusSelector  OutputSignals=position,params
  Data Type Conversion : DataTypeConversion  OutDataTypeStr=uint8  SaturateOnIntegerOverflow=off  RndMeth=Floor
  Lookahead Distance : Constant  Value=5  OutDataTypeStr=single
  Radius : Selector  InputPortWidth=4  IndexOptions=Index vector (dialog)  Indices=[3]  OutputSizes=1
  Relational Operator : RelationalOperator  Operator=>  OutDataTypeStr=boolean  RndMeth=Simplest  InputSameDT=off
  Sign : Signum  ZeroCross=off
  Terminator : Terminator
  Terminator1 : Terminator
  Turns : Selector  InputPortWidth=4  IndexOptions=Index vector (dialog)  Indices=[1]  OutputSizes=1
  UAV Orbit Follower : uavalgslib/Orbit Follower  UAVType=multirotor  MinOrbitRadius=1  MinLookaheadDistance=0.1  ExternalReset=none  ShowCrossTrackErrorOutput=off  ShowNumTurnsOutput=on  SimulateUsing=Code generation
  InnerLoopCmds : Outport  OutDataTypeStr=Bus: innerLoopCmdsBus
  Status : Outport  Port=2
  wires:
  Pose/1 -> UAV Orbit Follower/1
  Lookahead Distance/1 -> UAV Orbit Follower/5
  Abs/1 -> UAV Orbit Follower/3
  Bus Selector/1 -> UAV Orbit Follower/2  "<position>"
  ToWP/1 -> Bus Selector/1
  UAV Orbit Follower/1 -> Bus Creator/1  "LAP"
  Bus Creator/1 -> InnerLoopCmds/1
  UAV Orbit Follower/2 -> Bus Creator/2  "HeadingCmd"
  UAV Orbit Follower/3 -> Bus Creator/3  "YawCmd"
  Bus Selector/2 -> Turns/1, Radius/1  "<params>"
  Radius/1 -> Abs/1, Sign/1
  Sign/1 -> UAV Orbit Follower/4
  Relational Operator/1 -> Data Type Conversion/1
  Turns/1 -> Relational Operator/2
  Data Type Conversion/1 -> Status/1
  UAV Orbit Follower/6 -> Relational Operator/1
  UAV Orbit Follower/4 -> Terminator/1
  UAV Orbit Follower/5 -> Terminator1/1

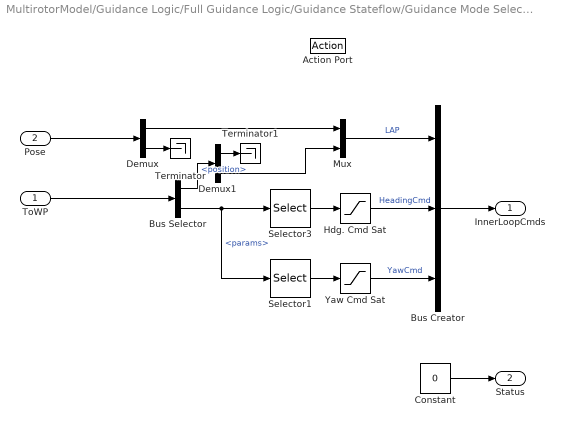
== system MultirotorModel/Guidance Logic/Full Guidance Logic/Guidance Stateflow/Guidance Mode Selector/GuidanceLogic.Takeoff ==
  ToWP : Inport
  Pose : Inport  Port=2
  Action Port : ActionPort
      settings: CopyFcn=Stateflow.SLINSF.SimulinkMan.removeBlockPreDeleteFcn  PreDeleteFcn=Stateflow.SLINSF.SimulinkMan.unsafePredeleteFcn
  Bus Creator : BusCreator  Inputs=3  OutDataTypeStr=Bus: innerLoopCmdsBus  NonVirtualBus=on
      settings: InheritFromInputs=off
  Bus Selector : BusSelector  OutputSignals=position,params
  Constant : Constant  Value=0  OutDataTypeStr=uint8
  Demux : Demux  Outputs=[2 2]
  Demux1 : Demux  Outputs=[2 1]
  Hdg. Cmd Sat : Saturate  UpperLimit=pi  LowerLimit=-pi
      settings: AttributesFormatString=[%<UpperLimit> %<LowerLimit>]
  Mux : Mux  Inputs=2
  Selector1 : Selector  InputPortWidth=4  IndexOptions=Index vector (dialog)  Indices=4  OutputSizes=1
  Selector3 : Selector  InputPortWidth=4  IndexOptions=Index vector (dialog)  Indices=4  OutputSizes=1
  Terminator : Terminator
  Terminator1 : Terminator
  Yaw Cmd Sat : Saturate  UpperLimit=pi  LowerLimit=-pi
      settings: AttributesFormatString=[%<UpperLimit> %<LowerLimit>]
  InnerLoopCmds : Outport  OutDataTypeStr=Bus: innerLoopCmdsBus
  Status : Outport  Port=2
  wires:
  Hdg. Cmd Sat/1 -> Bus Creator/2  "HeadingCmd"
  Bus Creator/1 -> InnerLoopCmds/1
  Constant/1 -> Status/1
  Pose/1 -> Demux/1
  Yaw Cmd Sat/1 -> Bus Creator/3  "YawCmd"
  ToWP/1 -> Bus Selector/1
  Bus Selector/2 -> Selector1/1, Selector3/1  "<params>"
  Mux/1 -> Bus Creator/1  "LAP"
  Demux/1 -> Mux/1
  Bus Selector/1 -> Demux1/1  "<position>"
  Demux1/2 -> Mux/2
  Demux/2 -> Terminator/1
  Demux1/1 -> Terminator1/1
  Selector3/1 -> Hdg. Cmd Sat/1
  Selector1/1 -> Yaw Cmd Sat/1

== system MultirotorModel/Guidance Logic/Full Guidance Logic/Guidance Stateflow/Guidance Mode Selector/GuidanceLogic.WP ==
  FromWP : Inport
  Pose : Inport  Port=2
  ToWP : Inport  Port=3
  Action Port : ActionPort
      settings: CopyFcn=Stateflow.SLINSF.SimulinkMan.removeBlockPreDeleteFcn  PreDeleteFcn=Stateflow.SLINSF.SimulinkMan.unsafePredeleteFcn
  APF_Avoidance : MATLAB Function  TreatAsAtomicUnit=on
  Bird : Constant  Value=[-119.5, -49.5, -15]
  Bus Creator : BusCreator  Inputs=3  OutDataTypeStr=Bus: innerLoopCmdsBus  NonVirtualBus=on
  Data Type Conversion : DataTypeConversion  OutDataTypeStr=uint8  SaturateOnIntegerOverflow=off  RndMeth=Floor
  Dist2WP : Subsystem
  Lookahead Distance : Constant  Value=15  OutDataTypeStr=single
  MATLAB Function : MATLAB Function  TreatAsAtomicUnit=on
  Relational Operator : RelationalOperator  OutDataTypeStr=boolean  RndMeth=Simplest  InputSameDT=off
  Scope : Scope
  Scope1 : Scope
  Waypoint Follower : uavalgslib/Waypoint Follower  UAVType=multirotor  StartFrom=closest  TransitionRadiusSource=internal  TransitionRadius=10  MinLookaheadDistance=0.1  HoverAtLastWaypoint=off  YawInput=on  ShowCrossTrackErrorOutput=off  ShowStatusOutput=off  SimulateUsing=Code generation
  InnerLoopCmds : Outport  OutDataTypeStr=Bus: innerLoopCmdsBus
  Status : Outport  Port=2
  wires:
  Data Type Conversion/1 -> Status/1
  Bus Creator/1 -> InnerLoopCmds/1
  ToWP/1 -> Dist2WP/3(ToWP), MATLAB Function/2(ToWP)
  Waypoint Follower/1 -> Bus Creator/1  "LAP"
  MATLAB Function/1(wps) -> Waypoint Follower/2
  Waypoint Follower/2 -> APF_Avoidance/2(desiredCourse)  "HeadingCmd"
  Waypoint Follower/3 -> APF_Avoidance/3(desiredYaw)  "YawCmd"
  Lookahead Distance/1 -> Relational Operator/1, Waypoint Follower/3
  Pose/1 -> Scope1/1, APF_Avoidance/1(pose), Waypoint Follower/1, Dist2WP/1(Pose)
  Waypoint Follower/4 -> Scope/1
  Dist2WP/1(Dist) -> Relational Operator/2
  FromWP/1 -> Dist2WP/2(FromWP), MATLAB Function/1(FromWP)
  Relational Operator/1 -> Data Type Conversion/1
  Bird/1 -> APF_Avoidance/4(obstacle)
  APF_Avoidance/1(correctedCourse) -> Bus Creator/2  "HeadingCmd"
  APF_Avoidance/2(correctedYaw) -> Bus Creator/3  "YawCmd"

== system MultirotorModel/Guidance Logic/Full Guidance Logic/Guidance Stateflow/UAV Path Manager ==
  In1 : Inport
  In3 : Inport  Port=2
  In4 : Inport  Port=3
  In5 : Inport  Port=4
  In2 : Inport  Port=5
  PathManagerSystemObject : MATLABSystem  System=uav.sluav.internal.system.PathManager  OutputBusName=uavPathManagerBus  DataType=single  UAVType=multirotor  LoiterRadius=LoiterRadius  SimulateUsing=Code generation
      mask Type: uav.sluav.internal.system.PathManager
      mask Display:
      | disp('PathManager');
      | port_label('input',1,'Pose');
      | port_label('input',2,'MissionData');
      | port_label('input',3,'isModeDone');
      | port_label('input',4,'MissionCmd');
      | port_label('input',5,'Home');
      | port_label('output',1,'ModeParams');
  Out1 : Outport
  wires:
  PathManagerSystemObject/1 -> Out1/1
  In1/1 -> PathManagerSystemObject/1
  In3/1 -> PathManagerSystemObject/2
  In4/1 -> PathManagerSystemObject/3
  In5/1 -> PathManagerSystemObject/4
  In2/1 -> PathManagerSystemObject/5

== system MultirotorModel/Guidance Logic/Obstacle Avoidance3D/Compute InnerLoop Cmds/FollowWaypoints ==
  UAVState : Inport
  GCSCmds : Inport  Port=2
  Atan2 : Trigonometry  Operator=atan2
  Bus Creator : BusCreator  Inputs=3  OutDataTypeStr=Bus: innerLoopCmdsBus  NonVirtualBus=on
  Bus Selector1 : BusSelector  OutputSignals=pos_vel.x,pos_vel.y,pos_vel.z,pos_vel.vy,pos_vel.vx
  Lookahead Distance : Constant  Value=4  OutDataTypeStr=single
  Mux : Mux
  Scope : Scope
  Scope1 : Scope
  Terminator : Terminator
  Waypoint Follower : uavalgslib/Waypoint Follower  UAVType=multirotor  StartFrom=first  TransitionRadiusSource=internal  TransitionRadius=0.5  MinLookaheadDistance=0.1  HoverAtLastWaypoint=off  YawInput=on  ShowCrossTrackErrorOutput=on  ShowStatusOutput=on  SimulateUsing=Code generation
  InnerLoopCmds : Outport  OutDataTypeStr=Bus: innerLoopCmdsBus
  wires:
  Bus Creator/1 -> InnerLoopCmds/1
  Bus Selector1/4 -> Atan2/1  "<vy>"
  Mux/1 -> Waypoint Follower/1
  Bus Selector1/2 -> Mux/2  "<y>"
  Waypoint Follower/6 -> Scope1/1
  Bus Selector1/3 -> Mux/3  "<z>"
  Bus Selector1/1 -> Mux/1  "<x>"
  Bus Selector1/5 -> Atan2/2  "<vx>"
  Waypoint Follower/2 -> Bus Creator/2  "HeadingCmd"
  Waypoint Follower/3 -> Bus Creator/3  "YawCmd"
  Waypoint Follower/5 -> Scope/1
  Lookahead Distance/1 -> Waypoint Follower/3
  Waypoint Follower/4 -> Terminator/1
  Atan2/1 -> Mux/4
  GCSCmds/1 -> Waypoint Follower/2
  Waypoint Follower/1 -> Bus Creator/1  "LAP"
  UAVState/1 -> Bus Selector1/1

== system MultirotorModel/Guidance Logic/Obstacle Avoidance3D/Compute InnerLoop Cmds/Hover ==
  In1 : Inport
  Bus Creator1 : BusCreator  Inputs=3  OutDataTypeStr=Bus: innerLoopCmdsBus  NonVirtualBus=on
  In2 : InportShadow
  In3 : InportShadow
  Selector : Selector  NumberOfDimensions=2  InputPortWidth=3  IndexOptions=Index vector (dialog),Index vector (dialog)  Indices=2,[1 2 3]  OutputSizes=1,1
  Selector1 : Selector  NumberOfDimensions=2  InputPortWidth=3  IndexOptions=Index vector (dialog),Index vector (dialog)  Indices=2,4  OutputSizes=1,1
  Selector2 : Selector  NumberOfDimensions=2  InputPortWidth=3  IndexOptions=Index vector (dialog),Index vector (dialog)  Indices=2,4  OutputSizes=1,1
  Transpose : Math  Operator=transpose
  Out1 : Outport
  wires:
  Selector/1 -> Transpose/1
  In3/1 -> Selector2/1
  In2/1 -> Selector1/1
  Selector2/1 -> Bus Creator1/3  "YawCmd"
  Bus Creator1/1 -> Out1/1
  Transpose/1 -> Bus Creator1/1  "LAP"
  Selector1/1 -> Bus Creator1/2  "HeadingCmd"
  In1/1 -> Selector/1

== system MultirotorModel/Guidance Logic/Obstacle Avoidance3D/Compute InnerLoop Cmds/Landing ==
  GCSCmds : Inport
  UAVState1 : Inport  Port=2  OutDataTypeStr=Bus: uavStateBus
  Atan1 : Trigonometry  Operator=atan2
  Bus Creator1 : BusCreator  Inputs=3  OutDataTypeStr=Bus: innerLoopCmdsBus  NonVirtualBus=on
  Bus Selector2 : BusSelector  OutputSignals=pos_vel.z,pos_vel.vy,pos_vel.vx
  Constant : Constant  Value=0  OutDataTypeStr=single
  Constant1 : Constant  Value=UAVSampleTime*4*4  OutDataTypeStr=single
  Mux1 : Mux  Inputs=2
  Saturation : Saturate  UpperLimit=-0.5  LowerLimit=-inf
  Selector : Selector  NumberOfDimensions=2  InputPortWidth=3  IndexOptions=Index vector (dialog),Index vector (dialog)  Indices=3,[1 2]  OutputSizes=1,1
  Sum : Sum
  Transpose : Math  Operator=transpose
  InnerLoopCmds1 : Outport  OutDataTypeStr=Bus: innerLoopCmdsBus
  wires:
  Mux1/1 -> Bus Creator1/1  "LAP"
  Bus Selector2/2 -> Atan1/1  "<vy>"
  Bus Selector2/3 -> Atan1/2  "<vx>"
  Atan1/1 -> Bus Creator1/2  "HeadingCmd"
  UAVState1/1 -> Bus Selector2/1
  Bus Creator1/1 -> InnerLoopCmds1/1
  GCSCmds/1 -> Selector/1
  Selector/1 -> Transpose/1
  Transpose/1 -> Mux1/1
  Constant/1 -> Bus Creator1/3  "YawCmd"
  Sum/1 -> Saturation/1
  Bus Selector2/1 -> Sum/2  "<z>"
  Constant1/1 -> Sum/1
  Saturation/1 -> Mux1/2

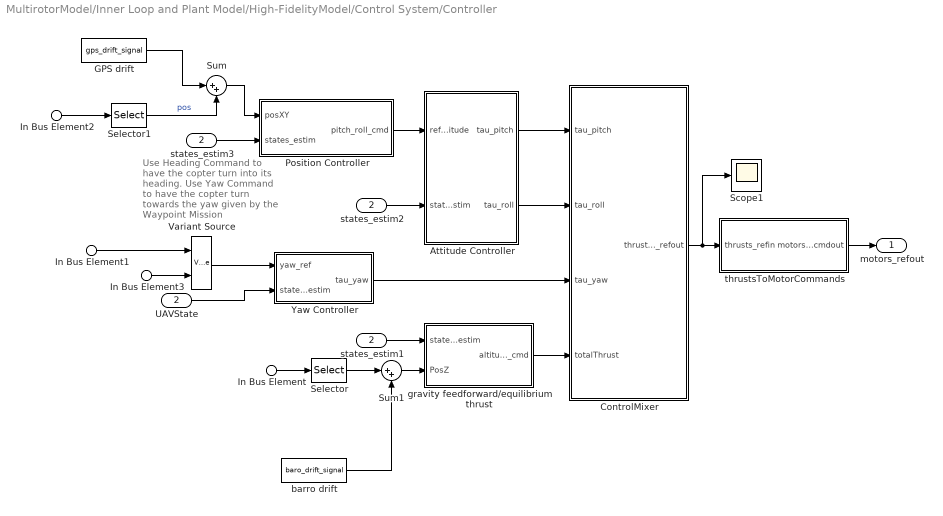
== system MultirotorModel/Inner Loop and Plant Model/High-FidelityModel/Control System/Controller ==
  note: Use Heading Command to have
      | the copter turn into its heading.
      | Use Yaw Command to have the
      | copter turn towards the yaw given
      | by the Waypoint Mission
  In Bus Element2 : Inport  PortName=PositionCmd  Element=LAP
  In Bus Element : Inport  PortName=PositionCmd  Element=LAP
  In Bus Element3 : Inport  PortName=PositionCmd  Element=YawCmd
  In Bus Element1 : Inport  PortName=PositionCmd  Element=HeadingCmd
  UAVState : Inport  Port=2
  Attitude Controller : Subsystem
  ControlMixer : Subsystem
  GPS drift : FromWorkspace  VariableName=gps_drift_signal  SampleTime=0.1
  Position Controller : Subsystem
  Scope1 : Scope
  Selector : Selector  InputPortWidth=3  IndexOptions=Index vector (dialog)  Indices=3  OutputSizes=1
  Selector1 : Selector  InputPortWidth=3  IndexOptions=Index vector (dialog)  Indices=[1 2]  OutputSizes=1
  Sum : Sum  Inputs=|++
  Sum1 : Sum  Inputs=|++
  Variant Source : VariantSource
  Yaw Controller : Subsystem
  barro drift : FromWorkspace  VariableName=baro_drift_signal  SampleTime=0.1
  gravity feedforward/equilibrium thrust : Subsystem
  states_estim1 : InportShadow  Port=2
  states_estim2 : InportShadow  Port=2
  states_estim3 : InportShadow  Port=2
  thrustsToMotorCommands : Subsystem
  motors_refout : Outport  VectorParamsAs1DForOutWhenUnconnected=off
  wires:
  thrustsToMotorCommands/1(motors_cmdout) -> motors_refout/1
  states_estim3/1 -> Position Controller/2(states_estim)
  ControlMixer/1(thrusts_refout) -> Scope1/1, thrustsToMotorCommands/1(thrusts_refin)
  gravity feedforward/equilibrium thrust/1(altitude_cmd) -> ControlMixer/4(totalThrust)
  states_estim1/1 -> gravity feedforward/equilibrium thrust/1(states_estim)
  UAVState/1 -> Yaw Controller/2(states_estim)
  states_estim2/1 -> Attitude Controller/2(states_estim)
  In Bus Element2/1 -> Selector1/1
  In Bus Element/1 -> Selector/1
  In Bus Element3/1 -> Variant Source/2
  Position Controller/1(pitch_roll_cmd) -> Attitude Controller/1(refAttitude)
  Variant Source/1 -> Yaw Controller/1(yaw_ref)
  In Bus Element1/1 -> Variant Source/1
  GPS drift/1 -> Sum/1
  Selector1/1 -> Sum/2  "pos"
  Sum/1 -> Position Controller/1(posXY)
  barro drift/1 -> Sum1/2
  Selector/1 -> Sum1/1
  Sum1/1 -> gravity feedforward/equilibrium thrust/2(PosZ)
  Attitude Controller/1(tau_pitch) -> ControlMixer/1(tau_pitch)
  Yaw Controller/1(tau_yaw) -> ControlMixer/3(tau_yaw)
  Attitude Controller/2(tau_roll) -> ControlMixer/2(tau_roll)

== system MultirotorModel/Inner Loop and Plant Model/High-FidelityModel/Plant Model/AC model ==
  Actuators : Inport
  Environment : Inport  Port=2
  DCM_be : Inport  Port=3
  V_b : Inport  Port=4  Unit=m/s
  w_b : Inport  Port=5  Unit=rad/s
  Applied Force Calculation : Subsystem
  Bus Selector : BusSelector  OutputSignals=Gravity_ned,AtmosphereBus.air_density
  Drag Calculation : Subsystem
  Gravity Force Calculation : Subsystem
  Motor Forces and Torques : Subsystem
  Scope4 : Scope
  Sum : Sum  Inputs=|+-
  Thrust Perterbation : Gain  Gain=ctrl_thrust_perturbation_param
  Vwind_b : Product  Multiplication=Matrix(*)
  wind : FromWorkspace  VariableName=wind_param  SampleTime=0.1
  F_cg : Outport  Unit=N  VectorParamsAs1DForOutWhenUnconnected=off
  M_cg : Outport  Port=2  Unit=N*m  VectorParamsAs1DForOutWhenUnconnected=off
  wires:
  Applied Force Calculation/1(External Forces) -> F_cg/1
  Motor Forces and Torques/2(Motor Torques) -> M_cg/1
  Bus Selector/1 -> Gravity Force Calculation/2(gravity)  "<Gravity_ned>"
  Gravity Force Calculation/1(gravity force) -> Applied Force Calculation/1(gravity force)
  Environment/1 -> Bus Selector/1
  Bus Selector/2 -> Motor Forces and Torques/2(Density), Drag Calculation/1(Density)  "<air_density>"
  DCM_be/1 -> Vwind_b/1, Gravity Force Calculation/1(DCMbe)
  Drag Calculation/1(Drag) -> Applied Force Calculation/2(Aerodynamic Forces)
  Actuators/1 -> Scope4/1, Motor Forces and Torques/4(Motor Commands)
  w_b/1 -> Motor Forces and Torques/3(pqr)
  Thrust Perterbation/1 -> Applied Force Calculation/3(Motor Forces)
  Motor Forces and Torques/1(Motor Forces) -> Thrust Perterbation/1
  wind/1 -> Vwind_b/2
  V_b/1 -> Sum/1
  Sum/1 -> Motor Forces and Torques/1(Vb), Drag Calculation/2(Vb)
  Vwind_b/1 -> Sum/2

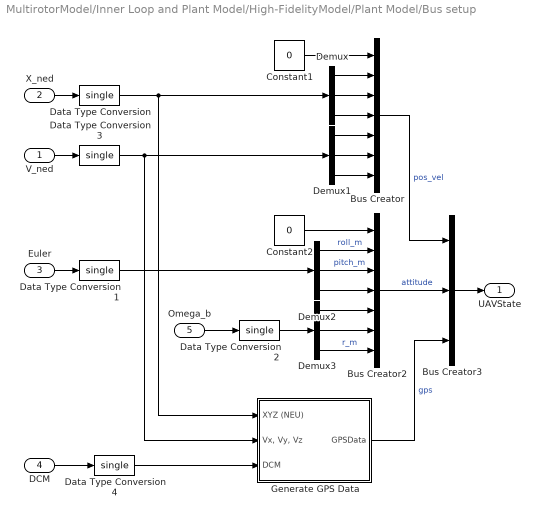
== system MultirotorModel/Inner Loop and Plant Model/High-FidelityModel/Plant Model/Bus setup ==
  V_ned : Inport  Unit=m/second  PortDimensions=3
  X_ned : Inport  Port=2  Unit=m  PortDimensions=3
  Euler : Inport  Port=3  Unit=rad  PortDimensions=3
  DCM : Inport  Port=4
  Omega_b : Inport  Port=5  Unit=rad/s  PortDimensions=3
  Bus Creator : BusCreator  Inputs=7  OutDataTypeStr=Bus: local_position_ned
      settings: InheritFromInputs=off
  Bus Creator2 : BusCreator  Inputs=7  OutDataTypeStr=Bus: attitudeBus
      settings: InheritFromInputs=off
  Bus Creator3 : BusCreator  Inputs=3  OutDataTypeStr=Bus: uavStateBus
      settings: InheritFromInputs=off
  Constant1 : Constant  Value=0  OutDataTypeStr=uint32
  Constant2 : Constant  Value=0  OutDataTypeStr=uint32
  Data Type Conversion{,1..4} (5 alike) : DataTypeConversion  OutDataTypeStr=single  SaturateOnIntegerOverflow=off  RndMeth=Floor
  Demux{,1..3} (4 alike) : Demux  Outputs=3
  Generate GPS Data : Subsystem
  UAVState : Outport  OutDataTypeStr=Bus: uavStateBus
  wires:
  Demux1/3 -> Bus Creator/7
  Bus Creator3/1 -> UAVState/1
  Demux/2 -> Bus Creator/3
  Demux3/2 -> Bus Creator2/6
  Bus Creator2/1 -> Bus Creator3/2  "attitude"
  Demux1/2 -> Bus Creator/6
  Demux3/1 -> Bus Creator2/5
  Demux/1 -> Bus Creator/2
  Euler/1 -> Data Type Conversion1/1
  Demux2/3 -> Bus Creator2/4
  Demux2/1 -> Bus Creator2/2  "roll_m"
  Bus Creator/1 -> Bus Creator3/1  "pos_vel"
  Constant2/1 -> Bus Creator2/1
  Demux2/2 -> Bus Creator2/3  "pitch_m"
  Demux3/3 -> Bus Creator2/7  "r_m"
  Demux1/1 -> Bus Creator/5
  V_ned/1 -> Data Type Conversion3/1
  Omega_b/1 -> Data Type Conversion2/1
  Demux/3 -> Bus Creator/4
  Constant1/1 -> Bus Creator/1
  Generate GPS Data/1(GPSData) -> Bus Creator3/3  "gps"
  X_ned/1 -> Data Type Conversion/1
  Data Type Conversion/1 -> Generate GPS Data/1(XYZ (NEU)), Demux/1
  Data Type Conversion2/1 -> Demux3/1
  Data Type Conversion1/1 -> Demux2/1
  Data Type Conversion3/1 -> Demux1/1, Generate GPS Data/2("Vx, Vy, Vz")
  DCM/1 -> Data Type Conversion4/1
  Data Type Conversion4/1 -> Generate GPS Data/3(DCM)
